simulink model "MicroMouseDebug"  (R2024a)
settings: Solver=VariableStepAuto  StartTime=0.0  StopTime=inf  FixedStep=0.001  RelTol=1e-3
model workspace (MAT data in the model file):
  comPort = "COM6"
  numBytes = Simulink.Parameter
  numBytes.Value = 5
  numBytes.Complexity = 'real'
  numBytes.Dimensions = [1 1]
  numBytes.DataType = 'auto'
libraries: etargetslib x47, instrumentseriallib x2, stmutilitieslib x1
settings Model: Creator=JesseJabezArendse  LastModifiedBy=user
settings DataIOCC: SaveOutput=off  SaveTime=off
settings OptimizationCC: DefaultParameterBehavior=Inlined  InlineInvariantSignals=on  EnhancedBackFolding=on  PassReuseOutputArgsAs=Individual arguments  StateBitsets=on  DataBitsets=on  ZeroExternalMemoryAtStartup=off  ZeroInternalMemoryAtStartup=off  NoFixptDivByZeroProtection=on  EfficientFloat2IntCast=on  OptimizeBlockOrder=speed  DifferentSizesBufferReuse=on  EfficientTunableParamExpr=on
settings DebuggingCC: ParameterPrecisionLossMsg=none  ParameterTunabilityLossMsg=error
settings SFSimCC: MATLABDynamicMemAlloc=off
settings RTWCC: Description=Embedded Coder  SystemTargetFile=ert.tlc  TemplateMakefile=ert_default_tmf  GenerateReport=on  RTWVerbose=off  IncludeHyperlinkInReport=on  LaunchReport=on  GenerateTraceInfo=on  GenerateTraceReport=on  GenerateTraceReportSl=on  GenerateTraceReportSf=on  GenerateTraceReportEml=on  GPUComputeCapability=3.5
settings CodeAppCC: ForceParamTrailComments=on  IgnoreCustomStorageClasses=off  OperatorAnnotations=on  SimulinkDataObjDesc=on  SFDataObjDesc=on  CustomSymbolStrGlobalVar=rt$N$M  CustomSymbolStrType=$N$M  CustomSymbolStrFcn=$N$M$F  CustomSymbolStrMacro=$N$M  InsertBlockDesc=on
settings ERTTargetCC: TargetLangStandard=C99 (ISO)  GenerateSampleERTMain=on  IncludeMdlTerminateFcn=off  CombineSignalStateStructs=on  PurelyIntegerCode=on  SupportNonFinite=off  InlinedParameterPlacement=NonHierarchical  ERTCustomFileTemplate=example_file_process.tlc

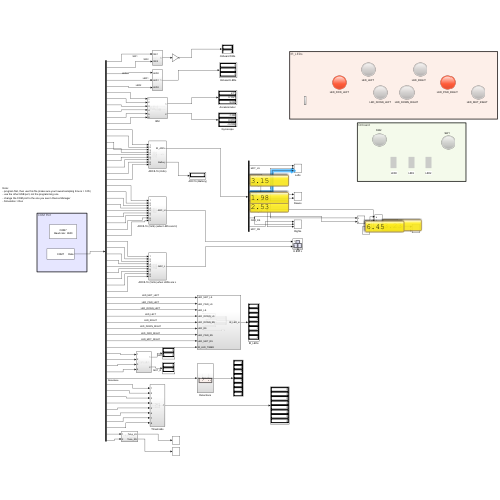
[thumbnail: Simulink's stored preview of the top-level diagram]
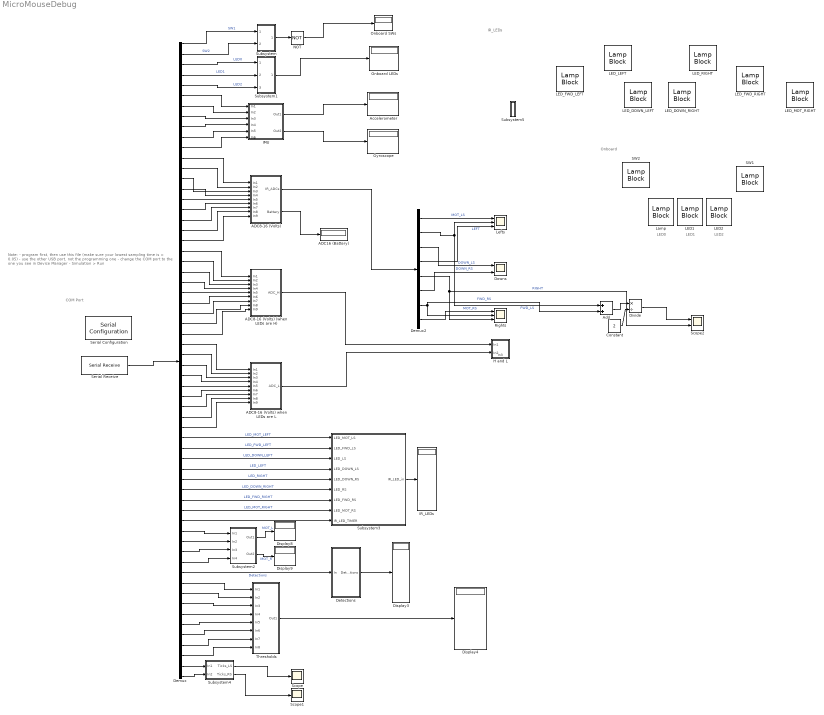
== system MicroMouseDebug ==
  note: Note:
      | - program first, then use this file (make sure your lowest sampling time is > 0.05)
      | - use the other USB port, not the programming one
      | - change the COM port to the one you see in Device Manager
      | - Simulation > Run
  note: Onboard
  note: LED0
  note: LED1
  note: LED2
  note: COM Port
  note: IR_LEDs
  ADC16 (Battery) : Display
  ADC8-16 (Volts) : Subsystem
  ADC8-16 (Volts) (when LEDs are H) : Subsystem
  ADC8-16 (Volts) when LEDs are L : Subsystem
  Accelerometer : Display
  Add : Sum
  Constant : Constant  Value=2
  Demux : Demux  Outputs=[1 1 1 1 1 4 4 4 4 4 4 2 2 2 2 2 2 2 2 2 2 2 2 2 2 2 2 2 2 2 2 2 2 2 2 2 2 2 1 1 1 1 1 1 1 1 4 2 2 2 2 8 2 2 2 2 2 2 2 2 4 4]
  Demux2 : Demux  Outputs=8
  Detections : Subsystem
  Display{3..4,8..9} (4 alike) : Display
  Divide : Product  Inputs=*/
  Downs : Scope  NumInputPorts=2
  Gyroscope : Display
  H and L : Subsystem
      settings: PortSchema="{\"entries\":[{\"content\":{\"sides\":[{\"content\":{\"connectorIds\":[\"In1\",\"In2\"]},\"type\":\"ConnectorPlacement.EquallySpacedRectSide\",\"uuid\":\"23d90d47-3dd1-43a3-8642-4eeff2833ca2\"},{\"content\":{\"side\":\"RIGHT\"},\"type\":\"ConnectorPlacement.EquallySpacedRectSide\",\"uuid\":\"72df7799-ca48-4914-91a2-cf4219a75fb9\"},{\"content\":{\"side\":\"TOP\"},\"type\":\"ConnectorPlacement.EquallySpacedRectSide\",\"uuid\":\"e5433b1e-26b9-4d31-8a79-7ab9e115cb00\"},{\"content\":{\"connectorIds\":[\"In3\"],\"side\":\"BOTTOM\"},\"type\":\"ConnectorPlacement.EquallySpacedRectSide\",\"uuid\":\"f8f19e1d-5eb6-4903-a782-b2a1368bb0bb\"}]},\"type\":\"ConnectorPlacement.EquallySpacedConnector\",\"uuid\":\"15bbc7f4-775b-4e52-896d-662c61b2b1c9\"}],\"packageUris\":[\"http://schema.mathworks.com/mf0/Connector/R2020b\"],\"version\":\"1.0\"}"
  IMU : Subsystem
  IR_LEDs : Display
  LED1 : LampBlock  LabelPosition=Hide  Icon=Rectangle
  LED2 : LampBlock  LabelPosition=Hide  Icon=Rectangle
  LED_DOWN_LEFT : LampBlock  LabelPosition=Hide
  LED_DOWN_RIGHT : LampBlock  LabelPosition=Hide
  LED_FWD_LEFT : LampBlock  LabelPosition=Hide
  LED_FWD_RIGHT : LampBlock  LabelPosition=Hide
  LED_LEFT : LampBlock  LabelPosition=Hide
  LED_MOT_RIGHT : LampBlock  LabelPosition=Hide
  LED_RIGHT : LampBlock  LabelPosition=Hide
  Lamp : LampBlock  LabelPosition=Hide  Icon=Rectangle
  Lefts : Scope  NumInputPorts=3
  NOT : Logic  Operator=NOT  IconShape=distinctive  AllPortsSameDT=off  OutDataTypeStr=boolean
  Onboard LEDs : Display
  Onboard SWs : Display
  Rights : Scope  NumInputPorts=3
  SW1 : LampBlock  LabelPosition=Hide
  SW2 : LampBlock  LabelPosition=Hide
  Scope : Scope
  Scope1 : Scope
  Scope2 : Scope  NumInputPorts=2
  Serial Configuration : instrumentseriallib/Serial Configuration  Priority=-200000  PortSel=COM7  Port=COM7  ComPort=COM7  BaudRate=9600  DataBits=8  Parity=none  StopBits=1  ByteOrder=little-endian  FlowControl=none  Timeout=10  SimulateUsing=Interpreted execution  BlockInModel=on  aMode=1
      settings: LibrarySourceBlock=embeddedtargetslib/Host Communication/Serial Configuration
  Serial Receive : instrumentseriallib/Serial Receive  Priority=1  PortSel=COM7  Port=COM7  ComPort=COM7  DataType=uint8  SaveDataType=uint8  ToggleHeader=on  Header='JJA'  ToggleDataSize=on  DataSize=[1 135]  ToggleTerminator=on  Terminator=Custom terminator  CustomTerminator='3099'  InputFormat=Column major  EnableBlockingMode=on  ActionDataUnavailable=Output last received value  ActionWhenDataUnavailable=Output last received value  CustomValue=0  SampleTime=0.1  SimulateUsing=Interpreted execution  BlockInModel=on  aMode=1
      settings: LibrarySourceBlock=embeddedtargetslib/Host Communication/Serial Receive
  Subsystem : Subsystem
  Subsystem1 : Subsystem
  Subsystem2 : Subsystem
  Subsystem3 : Subsystem
  Subsystem4 : Subsystem
  Subsystem5 : Subsystem
  Thresholds : Subsystem
  wires:
  Serial Receive/1 -> Demux/1
  Demux/12 -> ADC8-16 (Volts)/1(In1)
  Demux/13 -> ADC8-16 (Volts)/2(In2)
  Demux/14 -> ADC8-16 (Volts)/3(In3)
  Demux/15 -> ADC8-16 (Volts)/4(In4)
  Demux/16 -> ADC8-16 (Volts)/5(In5)
  Demux/17 -> ADC8-16 (Volts)/6(In6)
  Demux/18 -> ADC8-16 (Volts)/7(In7)
  Demux/19 -> ADC8-16 (Volts)/8(In8)
  Demux/20 -> ADC8-16 (Volts)/9(In9)
  Demux/6 -> IMU/1(In1)
  Demux/7 -> IMU/2(In2)
  Demux/8 -> IMU/3(In3)
  Demux/9 -> IMU/4(In4)
  Demux/10 -> IMU/5(In5)
  Demux/11 -> IMU/6(In6)
  IMU/1(Out1) -> Accelerometer/1
  IMU/2(Out2) -> Gyroscope/1
  Demux/1 -> Subsystem/1(SW1)  "SW1"
  Demux/2 -> Subsystem/2(SW2)  "SW2"
  Subsystem/1(Out1) -> NOT/1
  Demux/3 -> Subsystem1/1(LED0)  "LED0"
  Demux/4 -> Subsystem1/2(LED1)  "LED1"
  Demux/5 -> Subsystem1/3(LED2)  "LED2"
  Subsystem1/1(Out1) -> Onboard LEDs/1
  Demux/38 -> ADC8-16 (Volts) when LEDs are L/9(In9)
  Demux/37 -> ADC8-16 (Volts) when LEDs are L/8(In8)
  Demux/34 -> ADC8-16 (Volts) when LEDs are L/5(In5)
  Demux/33 -> ADC8-16 (Volts) when LEDs are L/4(In4)
  Demux/35 -> ADC8-16 (Volts) when LEDs are L/6(In6)
  Demux/32 -> ADC8-16 (Volts) when LEDs are L/3(In3)
  Demux/36 -> ADC8-16 (Volts) when LEDs are L/7(In7)
  Demux/31 -> ADC8-16 (Volts) when LEDs are L/2(In2)
  Demux/30 -> ADC8-16 (Volts) when LEDs are L/1(In1)
  Demux/29 -> ADC8-16 (Volts) (when LEDs are H)/9(In9)
  Demux/28 -> ADC8-16 (Volts) (when LEDs are H)/8(In8)
  Demux/25 -> ADC8-16 (Volts) (when LEDs are H)/5(In5)
  Demux/24 -> ADC8-16 (Volts) (when LEDs are H)/4(In4)
  Demux/26 -> ADC8-16 (Volts) (when LEDs are H)/6(In6)
  Demux/23 -> ADC8-16 (Volts) (when LEDs are H)/3(In3)
  Demux/27 -> ADC8-16 (Volts) (when LEDs are H)/7(In7)
  Demux/22 -> ADC8-16 (Volts) (when LEDs are H)/2(In2)
  Demux/21 -> ADC8-16 (Volts) (when LEDs are H)/1(In1)
  Demux/39 -> Subsystem3/1(LED_MOT_LS)  "LED_MOT_LEFT"
  Demux/40 -> Subsystem3/2(LED_FWD_LS)  "LED_FWD_LEFT"
  Demux/41 -> Subsystem3/3(LED_LS)  "LED_DOWN_LEFT"
  Demux/46 -> Subsystem3/8(LED_MOT_RS)  "LED_MOT_RIGHT"
  Demux/47 -> Subsystem3/9(IR_LED_TIMER)
  Subsystem2/2(Out2) -> Display9/1  "MOT_R"
  Demux/50 -> Subsystem2/3(In3)
  Demux/48 -> Subsystem2/1(In1)
  Demux/51 -> Subsystem2/4(In4)
  Subsystem2/1(Out1) -> Display8/1  "MOT_L"
  Demux/49 -> Subsystem2/2(In2)
  Demux/42 -> Subsystem3/4(LED_DOWN_LS)  "LED_LEFT"
  Demux/43 -> Subsystem3/5(LED_DOWN_RS)  "LED_RIGHT"
  Demux/44 -> Subsystem3/6(LED_RS)  "LED_DOWN_RIGHT"
  Demux/45 -> Subsystem3/7(LED_FWD_RS)  "LED_FWD_RIGHT"
  Demux2/1 -> Lefts/1  "MOT_LS"
  Demux2/2 -> Add/1, Lefts/2  "FWD_LS"
  Demux2/4 -> Lefts/3  "LEFT"
  Demux2/5 -> Scope2/2, Rights/3  "RIGHT"
  Demux2/7 -> Rights/2, Add/2  "FWD_RS"
  Demux2/8 -> Rights/1  "MOT_RS"
  Subsystem3/1(IR_LED_in) -> IR_LEDs/1
  NOT/1 -> Onboard SWs/1
  Demux/53 -> Thresholds/1(In1)
  Demux/54 -> Thresholds/2(In2)
  Demux/55 -> Thresholds/3(In3)
  Demux/56 -> Thresholds/4(In4)
  Demux/57 -> Thresholds/5(In5)
  Demux/58 -> Thresholds/6(In6)
  Demux/59 -> Thresholds/7(In7)
  Demux/60 -> Thresholds/8(In8)
  Demux2/3 -> Downs/1  "DOWN_LS"
  Demux2/6 -> Downs/2  "DOWN_RS"
  ADC8-16 (Volts)/2(Battery) -> ADC16 (Battery)/1
  ADC8-16 (Volts)/1(IR_ADCs) -> Demux2/1
  Demux/52 -> Detections/1(In)  "Detections"
  Detections/1(Detections) -> Display3/1
  Demux/61 -> Subsystem4/1(In1)
  Demux/62 -> Subsystem4/2(In2)
  Subsystem4/1(Ticks_LS) -> Scope/1
  Subsystem4/2(Ticks_RS) -> Scope1/1
  ADC8-16 (Volts) when LEDs are L/1(ADC_L) -> H and L/2(In2)
  ADC8-16 (Volts) (when LEDs are H)/1(ADC_H) -> H and L/1(In1)
  Thresholds/1(Out1) -> Display4/1
  Add/1 -> Divide/1
  Constant/1 -> Divide/2
  Divide/1 -> Scope2/1

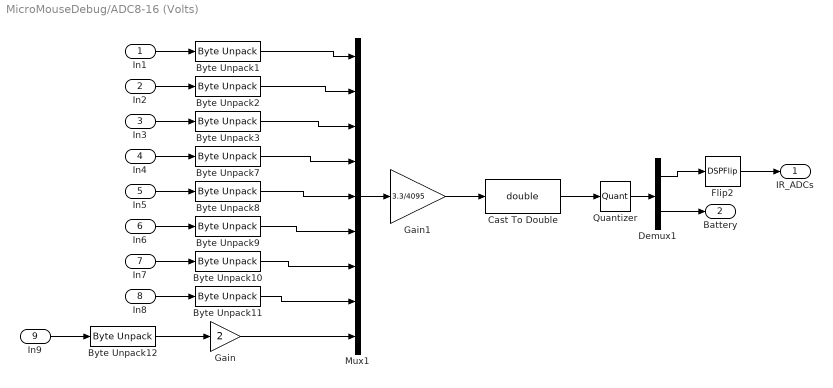
== system MicroMouseDebug/ADC8-16 (Volts) ==
  In1 : Inport
  In2 : Inport  Port=2
  In3 : Inport  Port=3
  In4 : Inport  Port=4
  In5 : Inport  Port=5
  In6 : Inport  Port=6
  In7 : Inport  Port=7
  In8 : Inport  Port=8
  In9 : Inport  Port=9
  Byte Unpack{1..3,7..12} (9 alike) : etargetslib/Byte Unpack  dimensions={[1]}  datatypes={'uint16'}  byteAlign=1
  Cast To Double : DataTypeConversion  OutDataTypeStr=double  SaturateOnIntegerOverflow=off  RndMeth=Floor
  Demux1 : Demux  Outputs=[8 1]
  Flip2 : DSPFlip
  Gain : Gain  Gain=2  OutDataTypeStr=uint16
  Gain1 : Gain  Gain=3.3/4095
  Mux1 : Mux  Inputs=9
  Quantizer : Quantizer  QuantizationInterval=0.01
  IR_ADCs : Outport
  Battery : Outport  Port=2
  wires:
  Cast To Double/1 -> Quantizer/1
  Gain/1 -> Mux1/9
  In9/1 -> Byte Unpack12/1
  In5/1 -> Byte Unpack8/1
  In7/1 -> Byte Unpack10/1
  In8/1 -> Byte Unpack11/1
  In4/1 -> Byte Unpack7/1
  In6/1 -> Byte Unpack9/1
  In1/1 -> Byte Unpack1/1
  In3/1 -> Byte Unpack3/1
  In2/1 -> Byte Unpack2/1
  Byte Unpack12/1 -> Gain/1
  Byte Unpack1/1 -> Mux1/1
  Byte Unpack11/1 -> Mux1/8
  Byte Unpack2/1 -> Mux1/2
  Byte Unpack8/1 -> Mux1/5
  Byte Unpack3/1 -> Mux1/3
  Byte Unpack7/1 -> Mux1/4
  Byte Unpack9/1 -> Mux1/6
  Byte Unpack10/1 -> Mux1/7
  Mux1/1 -> Gain1/1
  Gain1/1 -> Cast To Double/1
  Flip2/1 -> IR_ADCs/1
  Quantizer/1 -> Demux1/1
  Demux1/1 -> Flip2/1
  Demux1/2 -> Battery/1

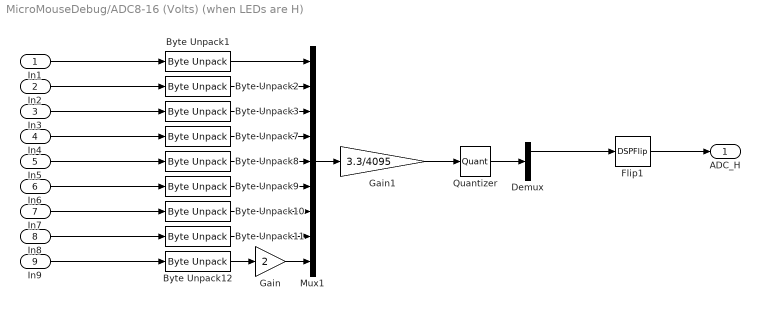
== system MicroMouseDebug/ADC8-16 (Volts) (when LEDs are H) ==
  In1 : Inport
  In2 : Inport  Port=2
  In3 : Inport  Port=3
  In4 : Inport  Port=4
  In5 : Inport  Port=5
  In6 : Inport  Port=6
  In7 : Inport  Port=7
  In8 : Inport  Port=8
  In9 : Inport  Port=9
  Byte Unpack{1..3,7..12} (9 alike) : etargetslib/Byte Unpack  dimensions={[1]}  datatypes={'uint16'}  byteAlign=1
  Demux : Demux  Outputs=[8 1]
  Flip1 : DSPFlip
  Gain : Gain  Gain=2  OutDataTypeStr=uint16
  Gain1 : Gain  Gain=3.3/4095  OutDataTypeStr=single
  Mux1 : Mux  Inputs=9
  Quantizer : Quantizer  QuantizationInterval=0.01
  ADC_H : Outport  OutDataTypeStr=single  PortDimensions=8
  wires:
  In7/1 -> Byte Unpack10/1
  Byte Unpack11/1 -> Mux1/8
  Byte Unpack8/1 -> Mux1/5
  Byte Unpack2/1 -> Mux1/2
  Byte Unpack12/1 -> Gain/1
  Byte Unpack7/1 -> Mux1/4
  In4/1 -> Byte Unpack7/1
  Byte Unpack1/1 -> Mux1/1
  In1/1 -> Byte Unpack1/1
  Gain/1 -> Mux1/9
  In6/1 -> Byte Unpack9/1
  Byte Unpack10/1 -> Mux1/7
  Byte Unpack9/1 -> Mux1/6
  Byte Unpack3/1 -> Mux1/3
  Mux1/1 -> Gain1/1
  Gain1/1 -> Quantizer/1
  In8/1 -> Byte Unpack11/1
  In3/1 -> Byte Unpack3/1
  In5/1 -> Byte Unpack8/1
  In2/1 -> Byte Unpack2/1
  In9/1 -> Byte Unpack12/1
  Demux/1 -> Flip1/1
  Quantizer/1 -> Demux/1
  Flip1/1 -> ADC_H/1

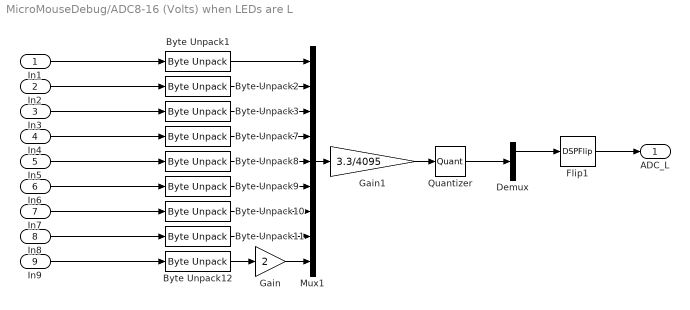
== system MicroMouseDebug/ADC8-16 (Volts) when LEDs are L ==
  In1 : Inport
  In2 : Inport  Port=2
  In3 : Inport  Port=3
  In4 : Inport  Port=4
  In5 : Inport  Port=5
  In6 : Inport  Port=6
  In7 : Inport  Port=7
  In8 : Inport  Port=8
  In9 : Inport  Port=9
  Byte Unpack{1..3,7..12} (9 alike) : etargetslib/Byte Unpack  dimensions={[1]}  datatypes={'uint16'}  byteAlign=1
  Demux : Demux  Outputs=[8 1]
  Flip1 : DSPFlip
  Gain : Gain  Gain=2  OutDataTypeStr=uint16
  Gain1 : Gain  Gain=3.3/4095  OutDataTypeStr=single
  Mux1 : Mux  Inputs=9
  Quantizer : Quantizer  QuantizationInterval=0.01
  ADC_L : Outport  OutDataTypeStr=single  PortDimensions=8
  wires:
  In7/1 -> Byte Unpack10/1
  Byte Unpack11/1 -> Mux1/8
  Byte Unpack8/1 -> Mux1/5
  Byte Unpack2/1 -> Mux1/2
  Byte Unpack12/1 -> Gain/1
  Byte Unpack7/1 -> Mux1/4
  In4/1 -> Byte Unpack7/1
  Byte Unpack1/1 -> Mux1/1
  In1/1 -> Byte Unpack1/1
  Gain/1 -> Mux1/9
  In6/1 -> Byte Unpack9/1
  Byte Unpack10/1 -> Mux1/7
  Byte Unpack9/1 -> Mux1/6
  Byte Unpack3/1 -> Mux1/3
  Mux1/1 -> Gain1/1
  In8/1 -> Byte Unpack11/1
  In3/1 -> Byte Unpack3/1
  In5/1 -> Byte Unpack8/1
  In2/1 -> Byte Unpack2/1
  In9/1 -> Byte Unpack12/1
  Gain1/1 -> Quantizer/1
  Demux/1 -> Flip1/1
  Quantizer/1 -> Demux/1
  Flip1/1 -> ADC_L/1

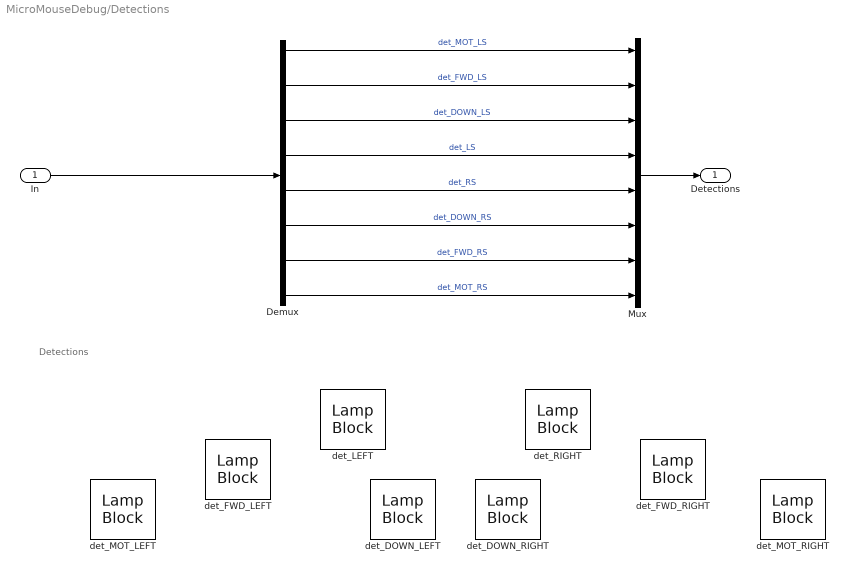
== system MicroMouseDebug/Detections ==
  note: Detections
  In : Inport
  Demux : Demux  Outputs=8
  Mux : Mux  Inputs=8
  det_DOWN_LEFT : LampBlock  LabelPosition=Hide
  det_DOWN_RIGHT : LampBlock  LabelPosition=Hide
  det_FWD_LEFT : LampBlock  LabelPosition=Hide
  det_FWD_RIGHT : LampBlock  LabelPosition=Hide
  det_LEFT : LampBlock  LabelPosition=Hide
  det_MOT_LEFT : LampBlock  LabelPosition=Hide
  det_MOT_RIGHT : LampBlock  LabelPosition=Hide
  det_RIGHT : LampBlock  LabelPosition=Hide
  Detections : Outport
  wires:
  In/1 -> Demux/1
  Demux/1 -> Mux/1  "det_MOT_LS"
  Demux/2 -> Mux/2  "det_FWD_LS"
  Demux/3 -> Mux/3  "det_DOWN_LS"
  Demux/4 -> Mux/4  "det_LS"
  Demux/5 -> Mux/5  "det_RS"
  Demux/6 -> Mux/6  "det_DOWN_RS"
  Demux/7 -> Mux/7  "det_FWD_RS"
  Demux/8 -> Mux/8  "det_MOT_RS"
  Mux/1 -> Detections/1

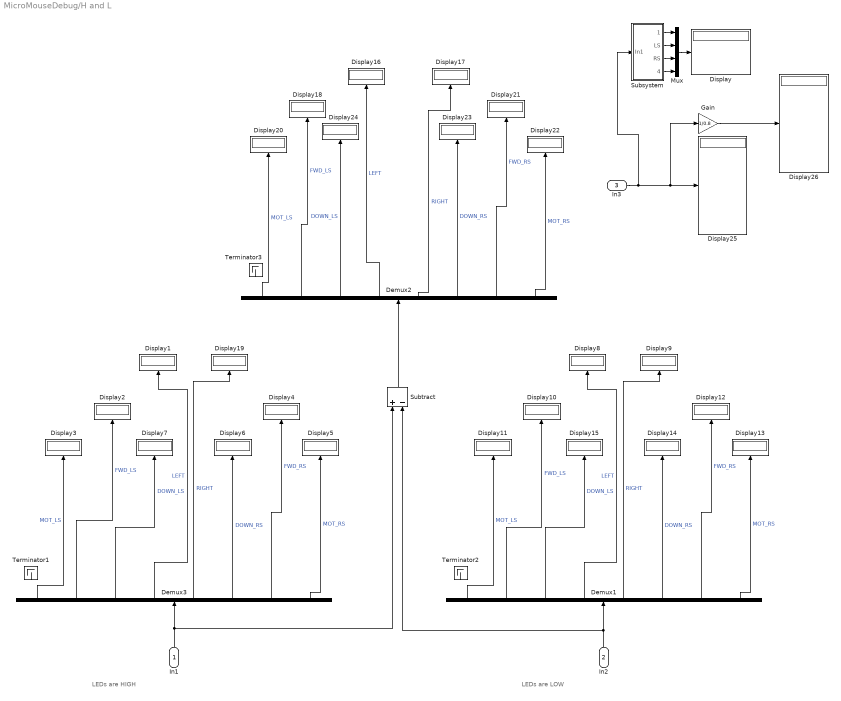
== system MicroMouseDebug/H and L ==
  note: LEDs are HIGH
  note: LEDs are LOW
  In1 : Inport
  In2 : Inport  Port=2
  In3 : Inport  Port=3
  Demux1 : Demux  Outputs=8
  Demux2 : Demux  Outputs=8
  Demux3 : Demux  Outputs=8
  Display{,1..26} (27 alike) : Display
      Display1 settings: Decimation=2
      Display10 settings: Decimation=2
      Display11 settings: Decimation=2
      Display12 settings: Decimation=2
      Display13 settings: Decimation=2
      Display14 settings: Decimation=2
      Display15 settings: Decimation=2
      Display16 settings: Decimation=2
      Display17 settings: Decimation=2
      Display18 settings: Decimation=2
      Display19 settings: Decimation=2
      Display2 settings: Decimation=2
      Display20 settings: Decimation=2
      Display21 settings: Decimation=2
      Display22 settings: Decimation=2
      Display23 settings: Decimation=2
      Display24 settings: Decimation=2
      Display3 settings: Decimation=2
      Display4 settings: Decimation=2
      Display5 settings: Decimation=2
      Display6 settings: Decimation=2
      Display7 settings: Decimation=2
      Display8 settings: Decimation=2
      Display9 settings: Decimation=2
  Gain : Gain  Gain=1/0.8
  Mux : Mux
  Subsystem : Subsystem
  Subtract : Sum  Inputs=+-  OutDataTypeStr=Inherit: Same as accumulator  AccumDataTypeStr=double  RndMeth=Nearest  SaturateOnIntegerOverflow=on
  Terminator1 : Terminator
  Terminator2 : Terminator
  Terminator3 : Terminator
  wires:
  Demux3/5 -> Display1/1  "LEFT"
  Demux3/2 -> Display4/1  "FWD_RS"
  Demux3/7 -> Display2/1  "FWD_LS"
  Demux3/4 -> Display19/1  "RIGHT"
  Demux3/8 -> Display3/1  "MOT_LS"
  Demux3/3 -> Display6/1  "DOWN_RS"
  Demux3/6 -> Display7/1  "DOWN_LS"
  Demux3/1 -> Display5/1  "MOT_RS"
  ? -> Terminator1/1
  In1/1 -> Demux3/1, Subtract/1
  Demux1/2 -> Display12/1  "FWD_RS"
  In2/1 -> Demux1/1, Subtract/2
  Demux1/1 -> Display13/1  "MOT_RS"
  Demux1/3 -> Display14/1  "DOWN_RS"
  Demux1/5 -> Display8/1  "LEFT"
  Demux1/8 -> Display11/1  "MOT_LS"
  Demux1/4 -> Display9/1  "RIGHT"
  Demux1/6 -> Display15/1  "DOWN_LS"
  ? -> Terminator2/1
  Demux1/7 -> Display10/1  "FWD_LS"
  Demux2/2 -> Display21/1  "FWD_RS"
  Demux2/1 -> Display22/1  "MOT_RS"
  Demux2/3 -> Display23/1  "DOWN_RS"
  Demux2/5 -> Display16/1  "LEFT"
  Demux2/8 -> Display20/1  "MOT_LS"
  Demux2/4 -> Display17/1  "RIGHT"
  Demux2/6 -> Display24/1  "DOWN_LS"
  ? -> Terminator3/1
  Demux2/7 -> Display18/1  "FWD_LS"
  Subtract/1 -> Demux2/1
  In3/1 -> Subsystem/1(In1), Gain/1, Display25/1
  Gain/1 -> Display26/1
  Subsystem/1(FWD_LS) -> Mux/1
  Subsystem/2(LS) -> Mux/2
  Subsystem/3(RS) -> Mux/3
  Subsystem/4(FWD_RS) -> Mux/4
  Mux/1 -> Display/1

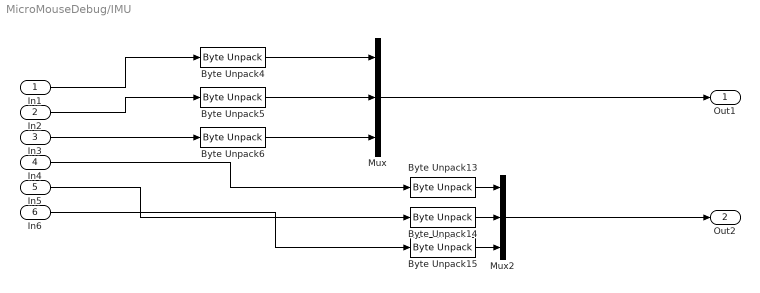
== system MicroMouseDebug/IMU ==
  In1 : Inport
  In2 : Inport  Port=2
  In3 : Inport  Port=3
  In4 : Inport  Port=4
  In5 : Inport  Port=5
  In6 : Inport  Port=6
  Byte Unpack{4..6,13..15} (6 alike) : etargetslib/Byte Unpack  dimensions={[1]}  datatypes={'single'}  byteAlign=1
  Mux : Mux  Inputs=3
  Mux2 : Mux  Inputs=3
  Out1 : Outport
  Out2 : Outport  Port=2
  wires:
  Byte Unpack4/1 -> Mux/1
  Byte Unpack14/1 -> Mux2/2
  Byte Unpack15/1 -> Mux2/3
  Mux2/1 -> Out2/1
  Byte Unpack13/1 -> Mux2/1
  In6/1 -> Byte Unpack15/1
  In3/1 -> Byte Unpack6/1
  Byte Unpack5/1 -> Mux/2
  Byte Unpack6/1 -> Mux/3
  In4/1 -> Byte Unpack13/1
  In1/1 -> Byte Unpack4/1
  In2/1 -> Byte Unpack5/1
  Mux/1 -> Out1/1
  In5/1 -> Byte Unpack14/1

== system MicroMouseDebug/Subsystem ==
  SW1 : Inport
  SW2 : Inport  Port=2
  Mux4 : Mux  Inputs=2
  Out1 : Outport
  wires:
  Mux4/1 -> Out1/1
  SW2/1 -> Mux4/2
  SW1/1 -> Mux4/1

== system MicroMouseDebug/Subsystem1 ==
  LED0 : Inport
  LED1 : Inport  Port=2
  LED2 : Inport  Port=3
  Mux3 : Mux  Inputs=3
  Out1 : Outport
  wires:
  Mux3/1 -> Out1/1
  LED2/1 -> Mux3/3
  LED0/1 -> Mux3/1
  LED1/1 -> Mux3/2

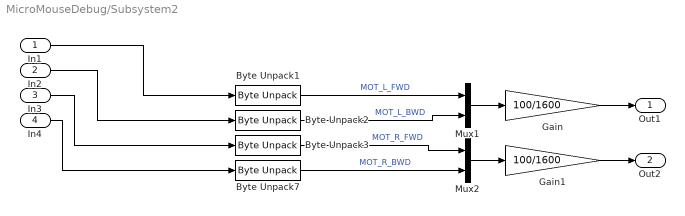
== system MicroMouseDebug/Subsystem2 ==
  In1 : Inport
  In2 : Inport  Port=2
  In3 : Inport  Port=3
  In4 : Inport  Port=4
  Byte Unpack{1..3,7} (4 alike) : etargetslib/Byte Unpack  dimensions={[1]}  datatypes={'uint16'}  byteAlign=1
  Gain : Gain  Gain=100/1600
  Gain1 : Gain  Gain=100/1600
  Mux1 : Mux  Inputs=2
  Mux2 : Mux  Inputs=2
  Out1 : Outport
  Out2 : Outport  Port=2
  wires:
  Byte Unpack2/1 -> Mux1/2  "MOT_L_BWD"
  In1/1 -> Byte Unpack1/1
  Byte Unpack3/1 -> Mux2/1  "MOT_R_FWD"
  Mux2/1 -> Gain1/1
  Byte Unpack7/1 -> Mux2/2  "MOT_R_BWD"
  Mux1/1 -> Gain/1
  Gain/1 -> Out1/1
  Byte Unpack1/1 -> Mux1/1  "MOT_L_FWD"
  In3/1 -> Byte Unpack3/1
  In2/1 -> Byte Unpack2/1
  In4/1 -> Byte Unpack7/1
  Gain1/1 -> Out2/1

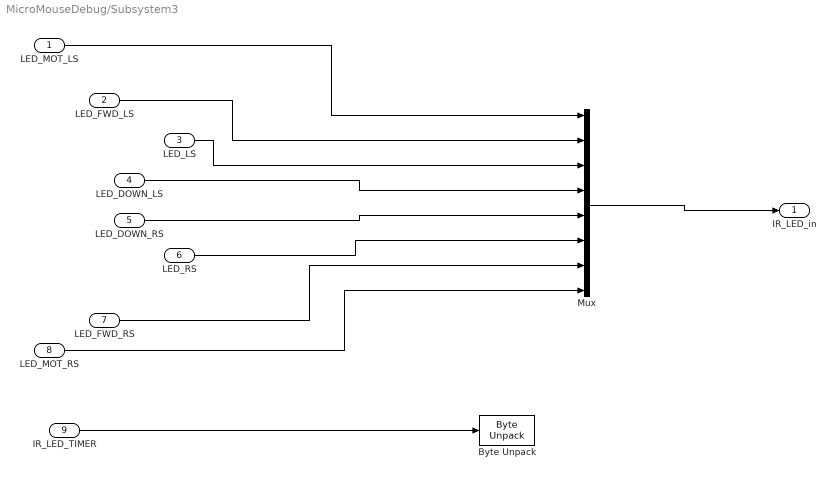
== system MicroMouseDebug/Subsystem3 ==
  LED_MOT_LS : Inport
  LED_FWD_LS : Inport  Port=2
  LED_LS : Inport  Port=3
  LED_DOWN_LS : Inport  Port=4
  LED_DOWN_RS : Inport  Port=5
  LED_RS : Inport  Port=6
  LED_FWD_RS : Inport  Port=7
  LED_MOT_RS : Inport  Port=8
  IR_LED_TIMER : Inport  Port=9
  Byte Unpack : stmutilitieslib/Byte Unpack  dimensions={[1]}  datatypes={'uint32'}  byteAlign=1  blockPlatform=stm32f4discovery
  Mux : Mux  Inputs=8
  IR_LED_in : Outport
  wires:
  IR_LED_TIMER/1 -> Byte Unpack/1
  Mux/1 -> IR_LED_in/1
  LED_FWD_LS/1 -> Mux/2
  LED_LS/1 -> Mux/3
  LED_MOT_LS/1 -> Mux/1
  LED_FWD_RS/1 -> Mux/7
  LED_MOT_RS/1 -> Mux/8
  LED_RS/1 -> Mux/6
  LED_DOWN_LS/1 -> Mux/4
  LED_DOWN_RS/1 -> Mux/5

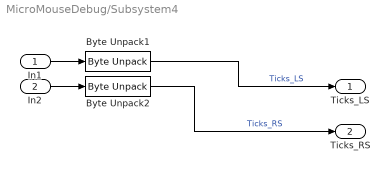
== system MicroMouseDebug/Subsystem4 ==
  In1 : Inport
  In2 : Inport  Port=2
  Byte Unpack1 : etargetslib/Byte Unpack  dimensions={[1]}  datatypes={'uint32'}  byteAlign=1
  Byte Unpack2 : etargetslib/Byte Unpack  dimensions={[1]}  datatypes={'uint32'}  byteAlign=1
  Ticks_LS : Outport
  Ticks_RS : Outport  Port=2
  wires:
  Byte Unpack2/1 -> Ticks_RS/1  "Ticks_RS"
  Byte Unpack1/1 -> Ticks_LS/1  "Ticks_LS"
  In2/1 -> Byte Unpack2/1
  In1/1 -> Byte Unpack1/1

== system MicroMouseDebug/Subsystem5 ==
  LED_MOT_LEFT : LampBlock  LabelPosition=Hide

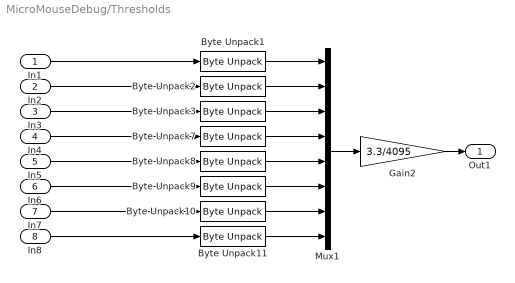
== system MicroMouseDebug/Thresholds ==
  In1 : Inport
  In2 : Inport  Port=2
  In3 : Inport  Port=3
  In4 : Inport  Port=4
  In5 : Inport  Port=5
  In6 : Inport  Port=6
  In7 : Inport  Port=7
  In8 : Inport  Port=8
  Byte Unpack{1..3,7..11} (8 alike) : etargetslib/Byte Unpack  dimensions={[1]}  datatypes={'uint16'}  byteAlign=1
  Gain2 : Gain  Gain=3.3/4095  OutDataTypeStr=single
  Mux1 : Mux  Inputs=8
  Out1 : Outport
  wires:
  Byte Unpack3/1 -> Mux1/3
  Byte Unpack8/1 -> Mux1/5
  Byte Unpack7/1 -> Mux1/4
  Mux1/1 -> Gain2/1
  Byte Unpack11/1 -> Mux1/8
  Byte Unpack9/1 -> Mux1/6
  Byte Unpack1/1 -> Mux1/1
  Byte Unpack10/1 -> Mux1/7
  Byte Unpack2/1 -> Mux1/2
  In5/1 -> Byte Unpack8/1
  In3/1 -> Byte Unpack3/1
  In4/1 -> Byte Unpack7/1
  In7/1 -> Byte Unpack10/1
  In8/1 -> Byte Unpack11/1
  In2/1 -> Byte Unpack2/1
  In6/1 -> Byte Unpack9/1
  In1/1 -> Byte Unpack1/1
  Gain2/1 -> Out1/1

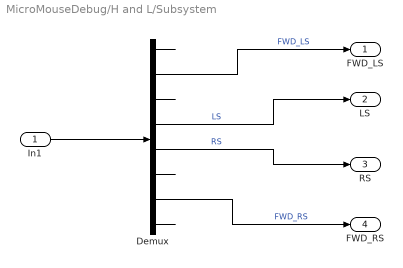
== system MicroMouseDebug/H and L/Subsystem ==
  In1 : Inport
  Demux : Demux  Outputs=8
  FWD_LS : Outport
  LS : Outport  Port=2
  RS : Outport  Port=3
  FWD_RS : Outport  Port=4
  wires:
  In1/1 -> Demux/1
  Demux/3 -> ?
  Demux/2 -> FWD_LS/1  "FWD_LS"
  Demux/1 -> ?
  Demux/6 -> ?
  Demux/8 -> ?
  Demux/7 -> FWD_RS/1  "FWD_RS"
  Demux/5 -> RS/1  "RS"
  Demux/4 -> LS/1  "LS"
